simulink model "position_control_PD_with_Due"  (R2021b)
settings: Solver=VariableStepAuto  StartTime=0.0  StopTime=10.0  RelTol=1e-3
undefined symbols (not defined in the file or in its folder): kd2, kp2
libraries: arduinolib x2
settings Model: Creator=DCLab  LastModifiedBy=DCLab

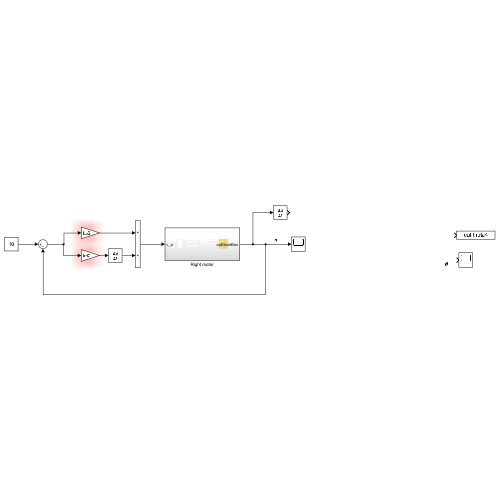
[thumbnail: Simulink's stored preview of the top-level diagram]
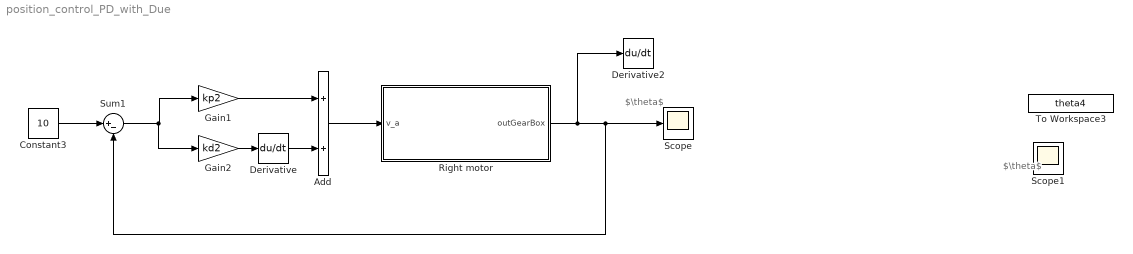
== system position_control_PD_with_Due ==
  note: $\theta$
  note: $\theta$
  Add : Sum
  Constant3 : Constant  Value=10
  Derivative : Derivative
  Derivative2 : Derivative
  Gain1 : Gain  Gain=kp2
  Gain2 : Gain  Gain=kd2
  Right motor : Subsystem
  Scope : Scope
  Scope1 : Scope
  Sum1 : Sum  Inputs=|+-
  To Workspace3 : ToWorkspace  VariableName=theta4  SampleTime=-1
      settings: Save2DSignal=2-D array (concatenate along first dimension)
  wires:
  Gain2/1 -> Derivative/1
  Sum1/1 -> Gain2/1, Gain1/1
  Derivative/1 -> Add/2
  Constant3/1 -> Sum1/1
  Gain1/1 -> Add/1
  Add/1 -> Right motor/1(v_a)
  Right motor/1(outGearBox) -> Sum1/2, Scope/1, Derivative2/1

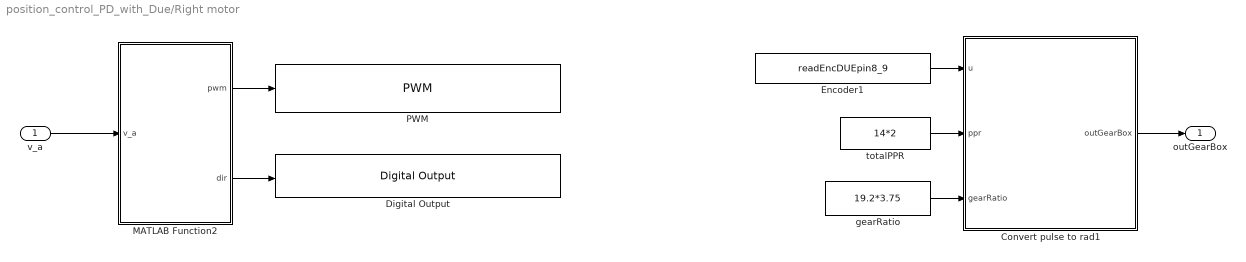
== system position_control_PD_with_Due/Right motor ==
  v_a : Inport
  Convert pulse to rad1 : MATLAB Function  TreatAsAtomicUnit=on
  Digital Output : arduinolib/Digital Output  pinNumber=7  Direction=output  blockPlatform=arduino
  Encoder1 : S-Function  InitFcn=try, set_param(gcb,'FunctionName','readEncDUEpin8_9'), end  FunctionName=readEncDUEpin8_9  SFunctionModules=readEncDUEpin8_9_wrapper  SFunctionDeploymentMode=off  EnableBusSupport=off  mask(S-Function Builder){}
      mask help: Simulink:masks:SFunctionBuilder_MD
      mask init:
      | val = [[.9  0.75 0.75 1 1 .9 .9 1]',[1 1 0.75 0.75 .9 .9 1 .9]'];try , sys = get_param(gcb,'SfunBuilderFcnName');if isempty(sys), sys = get_param(gcb,'FunctionName'); end,catch, sys = get_param(gcb,'FunctionName'); end
      settings: CopyFcn=set_param(gcbh,'LinkStatus','none')  PreSaveFcn=try, set_param(gcb,'FunctionName','readEncDUEpin8_9'), end  OpenFcn=sfunctionwizard(gcbh)
      mask Display:
      | plot(val(:,1),val(:,2))
      | disp(sys)
      | port_label('output',1,'count')
  MATLAB Function2 : MATLAB Function  TreatAsAtomicUnit=on
  PWM : arduinolib/PWM  pinNumber=6  frequencyType=Default  desiredFrequency=490.2  achievableFrequency=490.2
  gearRatio : Constant  Value=19.2*3.75
  totalPPR : Constant  Value=14*2
  outGearBox : Outport
  wires:
  totalPPR/1 -> Convert pulse to rad1/2(ppr)
  v_a/1 -> MATLAB Function2/1(v_a)
  MATLAB Function2/2(dir) -> Digital Output/1
  MATLAB Function2/1(pwm) -> PWM/1
  gearRatio/1 -> Convert pulse to rad1/3(gearRatio)
  Convert pulse to rad1/1(outGearBox) -> outGearBox/1
  Encoder1/1 -> Convert pulse to rad1/1(u)

== matlab function position_control_PD_with_Due/Right motor/MATLAB Function2 ==
  data: v_a input; pwm output; dir output
function [pwm,dir] = fcn(v_a)

vmax = 22.9;
pwm_cal = v_a*254/vmax;
if pwm_cal > 0
    pwm = pwm_cal;
    dir = 0;
elseif pwm_cal < 0
    pwm = abs(pwm_cal);
    dir = 1;
else
    pwm = 0;
    dir = 0;
end

== matlab function position_control_PD_with_Due/Right motor/Convert pulse to rad1 ==
  settings: updateMethod=DISCRETE
  data: u input; ppr input; gearRatio input; outGearBox output
function outGearBox = fcn(u,ppr,gearRatio)

persistent counter_num over_flag
if(isempty(counter_num)), counter_num = 0;end
if(isempty(over_flag)), over_flag = 0;end
pulse2radian = 2*pi/ppr; % 1 pulse = ?? radian

if(double(u) - counter_num > 40000), over_flag = over_flag-1;
elseif(double(u) - counter_num < -40000), over_flag = over_flag+1;
end

inGearBox = (double(u)+over_flag*(2^32 -1))*pulse2radian; 
outGearBox = inGearBox/gearRatio;
counter_num = double(u) ;
